simulink model "nonlinear_system"  (R2023a)
settings: Solver=VariableStepAuto  StartTime=0.0  StopTime=10.0  RelTol=1e-3
values from neighbouring files (symbols this model uses):
  Bl = 0    [ROBOT_CONTROL.m]    (also in collaborative_class_main.m)
  Bm = 0.015    [ROBOT_CONTROL.m]    (also in collaborative_class_main.m)
  g = 9.81    [ROBOT_CONTROL.m]    (also in collaborative_class_main.m)
  Jl = 4e-4    (= 0.0004)    [ROBOT_CONTROL.m]    (also in collaborative_class_main.m)
  Jm = 4e-4    (= 0.0004)    [ROBOT_CONTROL.m]    (also in collaborative_class_main.m)
  k = 0.8    [ROBOT_CONTROL.m]    (also in collaborative_class_main.m)
  l = 0.3    [ROBOT_CONTROL.m]    (also in collaborative_class_main.m)
  m = 0.3    [ROBOT_CONTROL.m]    (also in collaborative_class_main.m)
undefined symbols (not defined in the file or in its folder): x1, x2, x3, x4
settings Model: Creator=alexz  LastModifiedBy=alexz

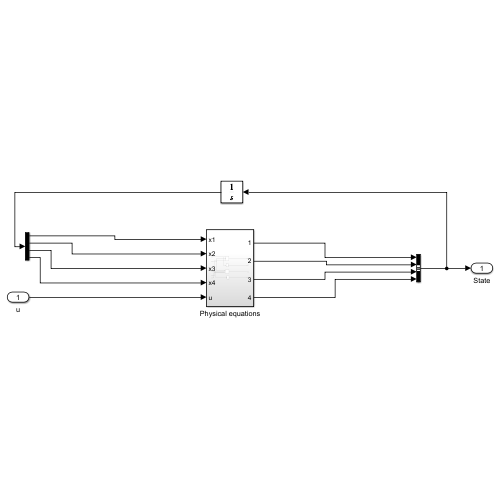
[thumbnail: Simulink's stored preview of the top-level diagram]
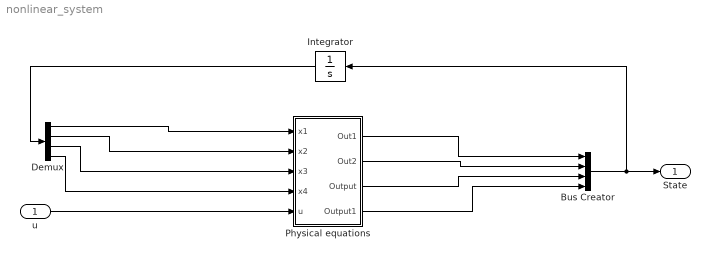
== system nonlinear_system ==
  u : Inport
  Bus Creator : BusCreator  Inputs=x1,x2,x3,x4
  Demux : Demux
  Integrator : Integrator
  Physical equations : Subsystem
  State : Outport
  wires:
  u/1 -> Physical equations/5(u)
  Physical equations/1(Out1) -> Bus Creator/1
  Physical equations/2(Out2) -> Bus Creator/2
  Physical equations/3(Output) -> Bus Creator/3
  Physical equations/4(Output1) -> Bus Creator/4
  Bus Creator/1 -> Integrator/1, State/1
  Integrator/1 -> Demux/1
  Demux/1 -> Physical equations/1(x1)
  Demux/2 -> Physical equations/2(x2)
  Demux/3 -> Physical equations/3(x3)
  Demux/4 -> Physical equations/4(x4)

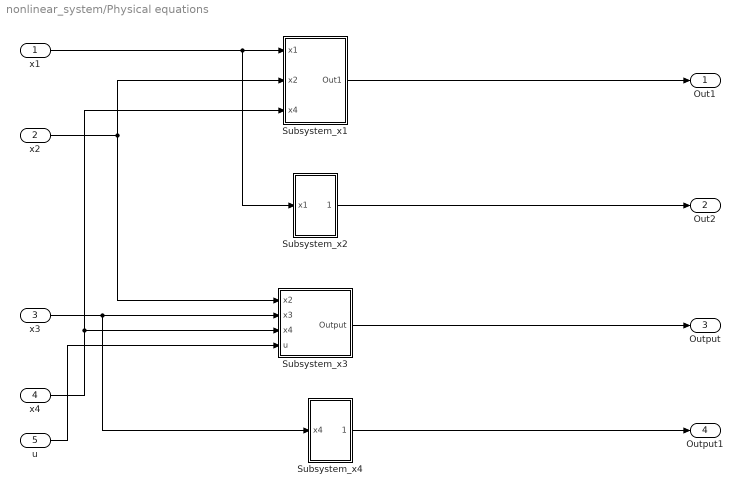
== system nonlinear_system/Physical equations ==
  x1 : Inport
  x2 : Inport  Port=2
  x3 : Inport  Port=3
  x4 : Inport  Port=4
  u : Inport  Port=5
  Subsystem_x1 : Subsystem
  Subsystem_x2 : Subsystem
  Subsystem_x3 : Subsystem
  Subsystem_x4 : Subsystem
  Out1 : Outport
  Out2 : Outport  Port=2
  Output : Outport  Port=3
  Output1 : Outport  Port=4
  wires:
  x1/1 -> Subsystem_x2/1(x1), Subsystem_x1/1(x1)
  x4/1 -> Subsystem_x3/3(x4), Subsystem_x1/3(x4)
  Subsystem_x3/1(Output) -> Output/1
  x3/1 -> Subsystem_x4/1(x4), Subsystem_x3/2(x3)
  x2/1 -> Subsystem_x3/1(x2), Subsystem_x1/2(x2)
  Subsystem_x4/1(Output) -> Output1/1
  Subsystem_x2/1(Out1) -> Out2/1
  Subsystem_x1/1(Out1) -> Out1/1
  u/1 -> Subsystem_x3/4(u)

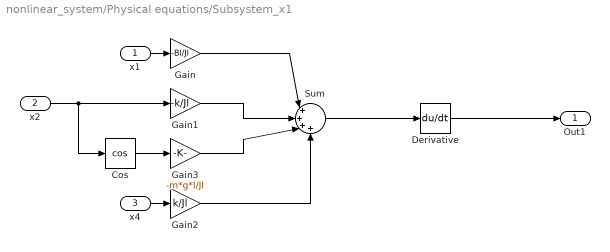
== system nonlinear_system/Physical equations/Subsystem_x1 ==
  x1 : Inport
  x2 : Inport  Port=2
  x4 : Inport  Port=3
  Cos : Trigonometry  Operator=cos
  Derivative : Derivative
  Gain : Gain  Gain=-Bl/Jl
  Gain1 : Gain  Gain=-k/Jl
  Gain2 : Gain  Gain=k/Jl
  Gain3 : Gain  Gain=-m*g*l/Jl
  Sum : Sum  Inputs=|++++
  Out1 : Outport
  wires:
  Sum/1 -> Derivative/1
  x1/1 -> Gain/1
  Gain3/1 -> Sum/3
  Gain1/1 -> Sum/2
  Gain/1 -> Sum/1
  Cos/1 -> Gain3/1
  Gain2/1 -> Sum/4
  Derivative/1 -> Out1/1
  x4/1 -> Gain2/1
  x2/1 -> Cos/1, Gain1/1

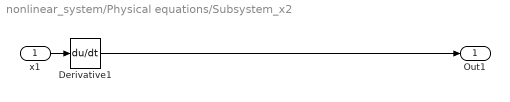
== system nonlinear_system/Physical equations/Subsystem_x2 ==
  x1 : Inport
  Derivative1 : Derivative
  Out1 : Outport
  wires:
  Derivative1/1 -> Out1/1
  x1/1 -> Derivative1/1

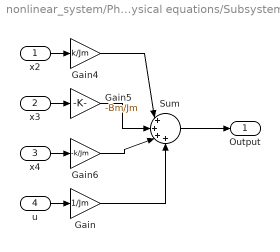
== system nonlinear_system/Physical equations/Subsystem_x3 ==
  x2 : Inport
  x3 : Inport  Port=2
  x4 : Inport  Port=3
  u : Inport  Port=4
  Gain : Gain  Gain=1/Jm
  Gain4 : Gain  Gain=k/Jm
  Gain5 : Gain  Gain=-Bm/Jm
  Gain6 : Gain  Gain=-k/Jm
  Sum : Sum  Inputs=|++++
  Output : Outport
  wires:
  x2/1 -> Gain4/1
  x4/1 -> Gain6/1
  x3/1 -> Gain5/1
  u/1 -> Gain/1
  Gain4/1 -> Sum/1
  Gain5/1 -> Sum/2
  Gain6/1 -> Sum/3
  Gain/1 -> Sum/4
  Sum/1 -> Output/1

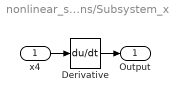
== system nonlinear_system/Physical equations/Subsystem_x4 ==
  x4 : Inport
  Derivative : Derivative
  Output : Outport
  wires:
  x4/1 -> Derivative/1
  Derivative/1 -> Output/1
